simulink model "IMM_UKF"  (R2012b)
settings: Solver=FixedStepDiscrete  StartTime=0.0  StopTime=SimulStop  FixedStep=0.05  RelTol=1e-3
undefined symbols (not defined in the file): mu1_init, mu2_init, PHI, SimulStop, T, T1, xhat_init
libraries: commnoisgen2 x1
settings Model: Creator=DonghanLee  LastModifiedBy=DonghanLee

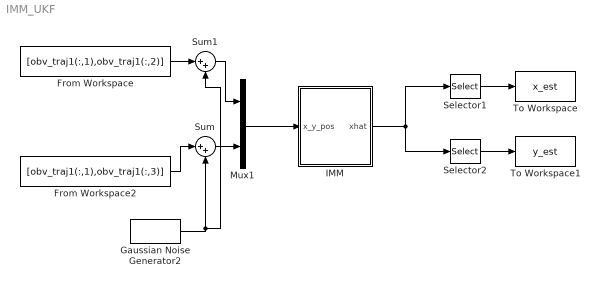
== system IMM_UKF ==
  From Workspace : FromWorkspace  VariableName=[obv_traj1(:,1),obv_traj1(:,2)]  SampleTime=0
  From Workspace2 : FromWorkspace  VariableName=[obv_traj1(:,1),obv_traj1(:,3)]  SampleTime=0
  Gaussian Noise Generator2 : commnoisgen2/Gaussian Noise Generator  m=0  d=noise  s=0  Ts=T  frameBased=off  sampPerFrame=1  orient=off  outDataType=double
  IMM : Subsystem
  Mux1 : Mux  Inputs=2
  Selector1 : Selector  InputPortWidth=5  IndexOptions=Index vector (dialog)  Indices=[1 2]  OutputSizes=1
  Selector2 : Selector  InputPortWidth=5  IndexOptions=Index vector (dialog)  Indices=[3 4]  OutputSizes=1
  Sum : Sum  Inputs=|++
  Sum1 : Sum  Inputs=|++
  To Workspace : ToWorkspace  VariableName=x_est  SampleTime=-1
  To Workspace1 : ToWorkspace  VariableName=y_est  SampleTime=-1
  wires:
  Mux1/1 -> IMM/1(x_y_pos)
  Gaussian Noise Generator2/1 -> Sum1/2, Sum/2
  From Workspace2/1 -> Sum/1
  Sum/1 -> Mux1/2
  From Workspace/1 -> Sum1/1
  Sum1/1 -> Mux1/1
  IMM/1(xhat) -> Selector2/1, Selector1/1
  Selector1/1 -> To Workspace/1
  Selector2/1 -> To Workspace1/1

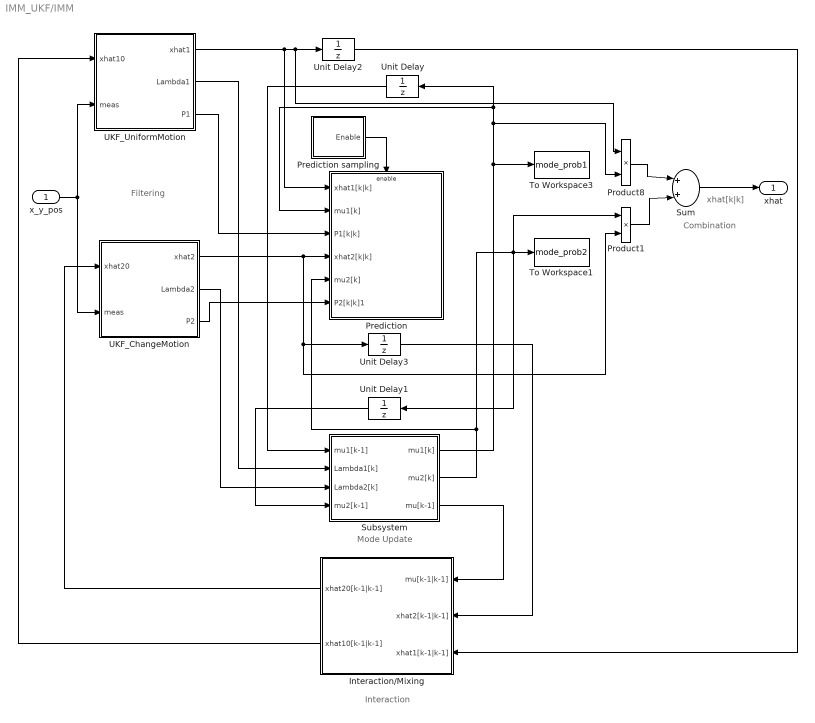
== system IMM_UKF/IMM ==
  note: Mode Update
  note: Interaction
  note: Filtering
  note: xhat[k|k]
  note: Combination
  x_y_pos : Inport
  Interaction/Mixing : Subsystem
  Prediction : Subsystem
  Prediction sampling : Subsystem
  Product1 : Product  SaturateOnIntegerOverflow=on  OutDataTypeStr=Inherit: Same as first input
  Product8 : Product  SaturateOnIntegerOverflow=on  OutDataTypeStr=Inherit: Same as first input
  Subsystem : Subsystem
  Sum : Sum  Inputs=|++|  SaturateOnIntegerOverflow=on
  To Workspace1 : ToWorkspace  VariableName=mode_prob2  SampleTime=-1
  To Workspace3 : ToWorkspace  VariableName=mode_prob1  SampleTime=-1
  UKF_ChangeMotion : Subsystem
  UKF_UniformMotion : Subsystem
  Unit Delay : UnitDelay  InitialCondition=mu1_init  SampleTime=-1
  Unit Delay1 : UnitDelay  InitialCondition=mu2_init  SampleTime=-1
  Unit Delay2 : UnitDelay  InitialCondition=xhat_init  SampleTime=-1
  Unit Delay3 : UnitDelay  InitialCondition=xhat_init  SampleTime=-1
  xhat : Outport
  wires:
  Product8/1 -> Sum/1
  Product1/1 -> Sum/2
  UKF_ChangeMotion/1(xhat2) -> Product1/2, Unit Delay3/1, Prediction/4(xhat2[k|k])
  Subsystem/3(mu[k-1]) -> Interaction/Mixing/1(mu[k-1|k-1])
  Interaction/Mixing/1(xhat20[k-1|k-1]) -> UKF_ChangeMotion/1(xhat20)
  Interaction/Mixing/2(xhat10[k-1|k-1]) -> UKF_UniformMotion/1(xhat10)
  Sum/1 -> xhat/1
  Unit Delay/1 -> Subsystem/1(mu1[k-1])
  Unit Delay1/1 -> Subsystem/4(mu2[k-1])
  Unit Delay3/1 -> Interaction/Mixing/2(xhat2[k-1|k-1])
  Unit Delay2/1 -> Interaction/Mixing/3(xhat1[k-1|k-1])
  x_y_pos/1 -> UKF_UniformMotion/2(meas), UKF_ChangeMotion/2(meas)
  UKF_UniformMotion/1(xhat1) -> Prediction/1(xhat1[k|k]), Product8/1, Unit Delay2/1
  UKF_UniformMotion/2(Lambda1) -> Subsystem/2(Lambda1[k])
  UKF_ChangeMotion/2(Lambda2) -> Subsystem/3(Lambda2[k])
  Subsystem/1(mu1[k]) -> To Workspace3/1, Product8/2, Unit Delay/1, Prediction/2("mu1[k] ")
  Subsystem/2(mu2[k]) -> Product1/1, To Workspace1/1, Unit Delay1/1, Prediction/5(mu2[k])
  Prediction sampling/1(Enable) -> Prediction/Enable
  UKF_UniformMotion/3(P1) -> Prediction/3(P1[k|k])
  UKF_ChangeMotion/3(P2) -> Prediction/6(P2[k|k]1)

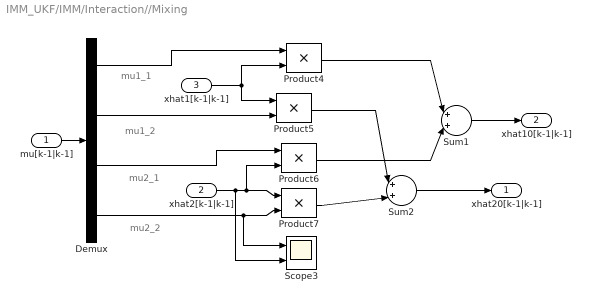
== system IMM_UKF/IMM/Interaction//Mixing ==
  note: mu1_1
  note: mu1_2
  note: mu2_1
  note: mu2_2
  mu[k-1|k-1] : Inport
  xhat2[k-1|k-1] : Inport  Port=2
  xhat1[k-1|k-1] : Inport  Port=3
  Demux : Demux
  Product{4..7} (4 alike) : Product  SaturateOnIntegerOverflow=on  OutDataTypeStr=Inherit: Same as first input
  Scope3 : Scope  NumInputPorts=2
      settings: TimeRange=10  YMin=-5~-5  YMax=5~5  SaveName=ScopeData7
  Sum1 : Sum  Inputs=|++|  SaturateOnIntegerOverflow=on
  Sum2 : Sum  Inputs=|++|  SaturateOnIntegerOverflow=on
  xhat20[k-1|k-1] : Outport
  xhat10[k-1|k-1] : Outport  Port=2
  wires:
  Demux/2 -> Product5/2
  Demux/4 -> Scope3/1, Product7/2
  Product4/1 -> Sum1/1
  Product6/1 -> Sum1/2
  xhat1[k-1|k-1]/1 -> Product4/2, Product5/1
  Demux/1 -> Product4/1
  Demux/3 -> Product6/1
  xhat2[k-1|k-1]/1 -> Scope3/2, Product6/2, Product7/1
  Product5/1 -> Sum2/1
  Product7/1 -> Sum2/2
  Sum2/1 -> xhat20[k-1|k-1]/1
  mu[k-1|k-1]/1 -> Demux/1
  Sum1/1 -> xhat10[k-1|k-1]/1

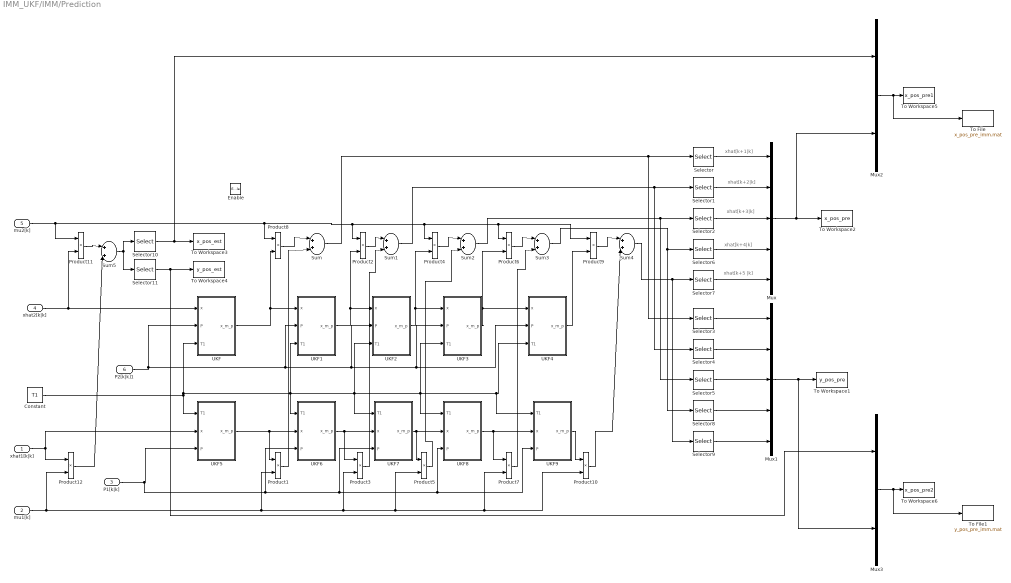
== system IMM_UKF/IMM/Prediction ==
  note: xhat[k+4|k]
  note: xhat[k+3|k]
  note: xhat[k+1|k]
  note: xhat[k+2|k]
  note: xhat[k+5 |k]
  xhat1[k|k] : Inport
  "mu1[k] " : Inport  Port=2
  P1[k|k] : Inport  Port=3
  xhat2[k|k] : Inport  Port=4
  mu2[k] : Inport  Port=5
  P2[k|k]1 : Inport  Port=6
  Enable : EnablePort
  Constant : Constant  Value=T1
  Mux : Mux  Inputs=5
  Mux1 : Mux  Inputs=5
  Mux2 : Mux  Inputs=2
  Mux3 : Mux  Inputs=2
  Product{1..12} (12 alike) : Product  SaturateOnIntegerOverflow=on  OutDataTypeStr=Inherit: Same as first input
  Selector{,1..2,6..7,10} (6 alike) : Selector  InputPortWidth=5  IndexOptions=Index vector (dialog)  Indices=[1]  OutputSizes=1
  Selector{3..5,8..9,11} (6 alike) : Selector  InputPortWidth=5  IndexOptions=Index vector (dialog)  Indices=[3]  OutputSizes=1
  Sum{,1..5} (6 alike) : Sum  Inputs=|++|  SaturateOnIntegerOverflow=on
  To File : ToFile  Filename=x_pos_pre_imm.mat  MatrixName=x_pos_pre_imm
  To File1 : ToFile  Filename=y_pos_pre_imm.mat  MatrixName=y_pos_pre_imm
  To Workspace1 : ToWorkspace  VariableName=y_pos_pre  SampleTime=-1
  To Workspace2 : ToWorkspace  VariableName=x_pos_pre  SampleTime=-1
  To Workspace3 : ToWorkspace  VariableName=x_pos_est  SampleTime=-1
  To Workspace4 : ToWorkspace  VariableName=y_pos_est  SampleTime=-1
  To Workspace5 : ToWorkspace  VariableName=x_pos_pre1  SampleTime=-1
  To Workspace6 : ToWorkspace  VariableName=x_pos_pre2  SampleTime=-1
  UKF : MATLAB Function  TreatAsAtomicUnit=on
  UKF1 : MATLAB Function  TreatAsAtomicUnit=on
  UKF2 : MATLAB Function  TreatAsAtomicUnit=on
  UKF3 : MATLAB Function  TreatAsAtomicUnit=on
  UKF4 : MATLAB Function  TreatAsAtomicUnit=on
  UKF5 : MATLAB Function  TreatAsAtomicUnit=on
  UKF6 : MATLAB Function  TreatAsAtomicUnit=on
  UKF7 : MATLAB Function  TreatAsAtomicUnit=on
  UKF8 : MATLAB Function  TreatAsAtomicUnit=on
  UKF9 : MATLAB Function  TreatAsAtomicUnit=on
  wires:
  xhat1[k|k]/1 -> UKF5/2(x), Product12/1
  UKF/1(x_m_p) -> Product8/2, UKF1/1(x)
  Product8/1 -> Sum/1
  UKF1/1(x_m_p) -> Product2/2, UKF2/1(x)
  Product2/1 -> Sum1/1
  UKF2/1(x_m_p) -> UKF3/1(x), Product4/2
  UKF7/1(x_m_p) -> UKF8/2(x), Product5/1
  Product4/1 -> Sum2/1
  Mux/1 -> Mux2/2, To Workspace2/1
  Mux1/1 -> Mux3/2, To Workspace1/1
  UKF5/1(x_m_p) -> Product1/1, UKF6/2(x)
  UKF6/1(x_m_p) -> Product3/1, UKF7/2(x)
  UKF3/1(x_m_p) -> UKF4/1(x), Product6/2
  UKF8/1(x_m_p) -> Product7/1, UKF9/2(x)
  Product6/1 -> Sum3/1
  mu2[k]/1 -> Product11/1, Product8/1, Product9/1, Product6/1, Product4/1, Product2/1
  "mu1[k] "/1 -> Product12/2, Product1/2, Product10/2, Product7/2, Product5/2, Product3/2
  UKF4/1(x_m_p) -> Product9/2
  UKF9/1(x_m_p) -> Product10/1
  Product9/1 -> Sum4/1
  Product10/1 -> Sum4/2
  Selector6/1 -> Mux/4
  Selector2/1 -> Mux/3
  Selector7/1 -> Mux/5
  Selector/1 -> Mux/1
  Selector1/1 -> Mux/2
  Selector3/1 -> Mux1/1
  Selector4/1 -> Mux1/2
  Selector5/1 -> Mux1/3
  Selector8/1 -> Mux1/4
  Selector9/1 -> Mux1/5
  Sum/1 -> Selector/1, Selector3/1
  Sum1/1 -> Selector4/1, Selector1/1
  Sum2/1 -> Selector5/1, Selector2/1
  Sum3/1 -> Selector8/1, Selector6/1
  Sum4/1 -> Selector9/1, Selector7/1
  xhat2[k|k]/1 -> Product11/2, UKF/1(x)
  Product11/1 -> Sum5/1
  Product12/1 -> Sum5/2
  Sum5/1 -> Selector11/1, Selector10/1
  Selector10/1 -> Mux2/1, To Workspace3/1
  Selector11/1 -> Mux3/1, To Workspace4/1
  Mux2/1 -> To File/1, To Workspace5/1
  Mux3/1 -> To Workspace6/1, To File1/1
  P2[k|k]1/1 -> UKF/2(P), UKF1/2(P), UKF2/2(P), UKF4/2(P), UKF3/2(P)
  Constant/1 -> UKF6/1(T1), UKF7/1(T1), UKF8/1(T1), UKF3/3(T1), UKF9/1(T1), UKF4/3(T1), UKF2/3(T1), UKF1/3(T1), UKF/3(T1), UKF5/1(T1)
  P1[k|k]/1 -> UKF8/3(P), UKF9/3(P), UKF7/3(P), UKF6/3(P), UKF5/3(P)
  Product1/1 -> Sum/2
  Product3/1 -> Sum1/2
  Product5/1 -> Sum2/2
  Product7/1 -> Sum3/2

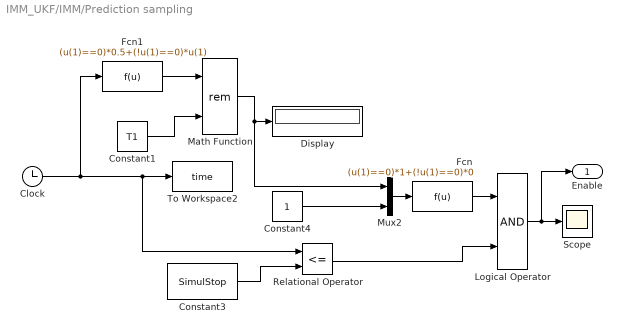
== system IMM_UKF/IMM/Prediction sampling ==
  Clock : Clock
  Constant1 : Constant  Value=T1
  Constant3 : Constant  Value=SimulStop
  Constant4 : Constant
  Display : Display
  Fcn : Fcn  Expr=(u(1)==0)*1+(!u(1)==0)*0
  Fcn1 : Fcn  Expr=(u(1)==0)*0.5+(!u(1)==0)*u(1)
  Logical Operator : Logic  AllPortsSameDT=off  OutDataTypeStr=boolean
  Math Function : Math  Operator=rem  SaturateOnIntegerOverflow=on
  Mux2 : Mux  Inputs=2
  Relational Operator : RelationalOperator  Operator=<=  OutDataTypeStr=boolean
  Scope : Scope
      settings: SaveName=ScopeData2
  To Workspace2 : ToWorkspace  VariableName=time  SampleTime=-1
  Enable : Outport
  wires:
  Clock/1 -> Fcn1/1, Relational Operator/1, To Workspace2/1
  Constant1/1 -> Math Function/2
  Math Function/1 -> Mux2/1, Display/1
  Logical Operator/1 -> Enable/1, Scope/1
  Fcn/1 -> Logical Operator/1
  Relational Operator/1 -> Logical Operator/2
  Constant3/1 -> Relational Operator/2
  Constant4/1 -> Mux2/2
  Mux2/1 -> Fcn/1
  Fcn1/1 -> Math Function/1

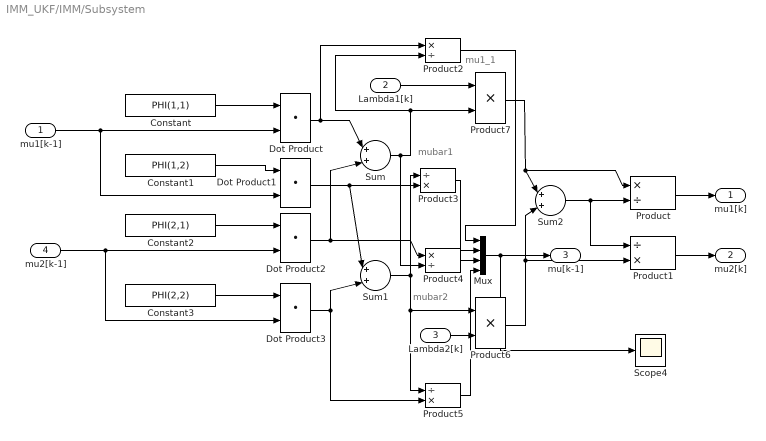
== system IMM_UKF/IMM/Subsystem ==
  note: mubar1
  note: mubar2
  note: mu1_1
  mu1[k-1] : Inport
  Lambda1[k] : Inport  Port=2
  Lambda2[k] : Inport  Port=3
  mu2[k-1] : Inport  Port=4
  Constant : Constant  Value=PHI(1,1)
  Constant1 : Constant  Value=PHI(1,2)
  Constant2 : Constant  Value=PHI(2,1)
  Constant3 : Constant  Value=PHI(2,2)
  Dot Product{,1..3} (4 alike) : DotProduct  InputSameDT=on  OutDataTypeStr=Inherit: Inherit via internal rule
  Mux : Mux
  Product : Product  Inputs=*/  SaturateOnIntegerOverflow=on  OutDataTypeStr=Inherit: Same as first input
  Product1 : Product  Inputs=/*  SaturateOnIntegerOverflow=on  OutDataTypeStr=Inherit: Same as first input
  Product2 : Product  Inputs=*/  SaturateOnIntegerOverflow=on  OutDataTypeStr=Inherit: Same as first input
  Product3 : Product  Inputs=/*  SaturateOnIntegerOverflow=on  OutDataTypeStr=Inherit: Same as first input
  Product4 : Product  Inputs=*/  SaturateOnIntegerOverflow=on  OutDataTypeStr=Inherit: Same as first input
  Product5 : Product  Inputs=/*  SaturateOnIntegerOverflow=on  OutDataTypeStr=Inherit: Same as first input
  Product6 : Product  SaturateOnIntegerOverflow=on  OutDataTypeStr=Inherit: Same as first input
  Product7 : Product  SaturateOnIntegerOverflow=on  OutDataTypeStr=Inherit: Same as first input
  Scope4 : Scope
      settings: YMin=2.77556e-17  YMax=1  SaveName=ScopeData31
  Sum : Sum  Inputs=|++|  SaturateOnIntegerOverflow=on
  Sum1 : Sum  Inputs=|++|  SaturateOnIntegerOverflow=on
  Sum2 : Sum  Inputs=|++|  SaturateOnIntegerOverflow=on
  mu1[k] : Outport
  mu2[k] : Outport  Port=2
  mu[k-1] : Outport  Port=3
  wires:
  Constant/1 -> Dot Product/1
  Constant1/1 -> Dot Product1/1
  Constant2/1 -> Dot Product2/1
  Constant3/1 -> Dot Product3/1
  mu1[k-1]/1 -> Dot Product/2, Dot Product1/2
  mu2[k-1]/1 -> Dot Product2/2, Dot Product3/2
  Dot Product/1 -> Sum/1, Product2/1
  Dot Product2/1 -> Sum/2, Product4/1
  Dot Product1/1 -> Sum1/1, Product3/2
  Dot Product3/1 -> Sum1/2, Product5/2
  Sum1/1 -> Product5/1, Product6/1, Product3/1
  Sum/1 -> Product2/2, Product7/2, Product4/2
  Lambda1[k]/1 -> Product7/1
  Lambda2[k]/1 -> Product6/2
  Product7/1 -> Sum2/1, Product/1
  Product6/1 -> Sum2/2, Product1/2
  Sum2/1 -> Product/2, Product1/1
  Product/1 -> mu1[k]/1
  Product1/1 -> mu2[k]/1
  Product4/1 -> Mux/3
  Product2/1 -> Mux/1
  Product3/1 -> Mux/2
  Product5/1 -> Mux/4
  Mux/1 -> mu[k-1]/1, Scope4/1

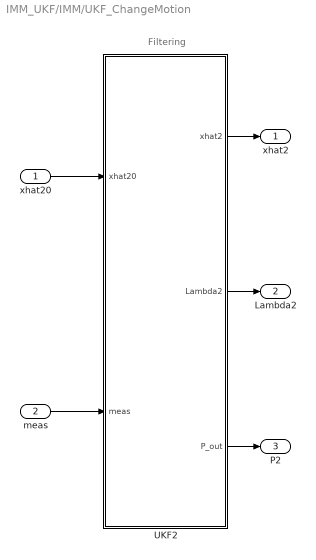
== system IMM_UKF/IMM/UKF_ChangeMotion ==
  note: Filtering
  xhat20 : Inport
  meas : Inport  Port=2
  UKF2 : MATLAB Function  TreatAsAtomicUnit=on
  xhat2 : Outport
  Lambda2 : Outport  Port=2
  P2 : Outport  Port=3
  wires:
  UKF2/2(Lambda2) -> Lambda2/1
  UKF2/1(xhat2) -> xhat2/1
  xhat20/1 -> UKF2/1(xhat20)
  meas/1 -> UKF2/2(meas)
  UKF2/3(P_out) -> P2/1

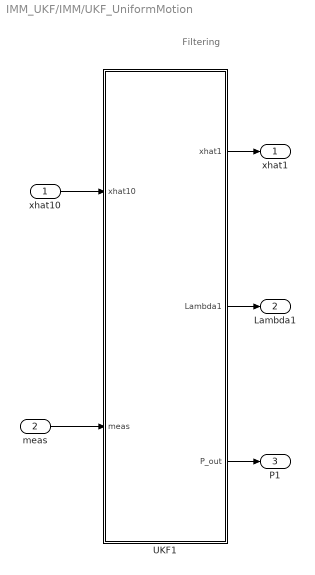
== system IMM_UKF/IMM/UKF_UniformMotion ==
  note: Filtering
  xhat10 : Inport
  meas : Inport  Port=2
  UKF1 : MATLAB Function  TreatAsAtomicUnit=on
  xhat1 : Outport
  Lambda1 : Outport  Port=2
  P1 : Outport  Port=3
  wires:
  meas/1 -> UKF1/2(meas)
  xhat10/1 -> UKF1/1(xhat10)
  UKF1/1(xhat1) -> xhat1/1
  UKF1/2(Lambda1) -> Lambda1/1
  UKF1/3(P_out) -> P1/1

== matlab function IMM_UKF/IMM/UKF_UniformMotion/UKF1 ==
  data: xhat10 input; meas input; xhat1 output; Lambda1 output; P_out output
function [xhat1,Lambda1,P_out] = UKF1(xhat10,meas)
% Define parametersInitialization
T=0.05; % Sampling time [s]
L=5; % Dimension of state vector
% Scaling Factors & Weights
alpha=0.001;                                 %default, tunable
kappa=0;                                       %default, tunable
beta=2;                                     %default, tunable

lambda=alpha^2*(L+kappa)-L;                    %scaling factor
c=L+lambda;                                 %scaling factor
% Wm=[lambda/c 0.5/c*ones(1,2*L)];           %weights for means
% Wc=Wm;
% Wc(1)=Wc(1)+(1-alpha^2+beta);               %weights for covariance

Wm = ones(2*L + 1,1)*1/(2*(L+lambda));
Wc = Wm;
Wm(1) = lambda/(lambda+L);
Wc(1) = lambda/(lambda+L) + 1 - alpha^2 + beta;
c=sqrt(c);

H = [1 0 0 0 0;
     0 0 1 0 0];

% Initialize
persistent P1 W1 V1
if isempty(P1)

% meas_noise1 = 0.5; 
% a_process_noise = 5*10^(-3); 
% w_process_noise = 5*10^(-3);     

% New Feezed value
meas_noise1 = 1.5; 
a_process_noise = 1.5*10^(-2); 
w_process_noise = 1.5*10^(-2);  

Sv1 = meas_noise1^2;
Sw1 = a_process_noise^2;
Sw2 = w_process_noise^2;
Sw = [Sw1 0 0;0 Sw1 0;0 0 Sw2];
%Bw = [0.5*T^2 0 0;T 0 0;0 0.5*T^2 0;0 T 0;0 0 T];

Bw = [T 0 0;1 0 0;0 T 0;0 1 0;0 0 1];

Dw = eye(2);
W1 = Bw*Sw*Bw';
V1 = Dw*Sv1*Dw';

P1 = eye(5,5);
% x = zeros(L, 2*L+1);
% x(:,1) = [meas(1,1);10^(-5);meas(2,1);0;10^(-5)];
%x(:,1) = [meas(1,1);10;meas(2,1);0;10^(-5)];

%y = zeros(L, 2*L+1);
end
% Generate sigma points
x=xhat10;
sP = chol(P1,'lower');
chi_p = [x(:,1) x(:,1)*ones(1,L)+c*sP x(:,1)*ones(1,L)-c*sP];

% Prediction 
    chi_m = zeros(L,2*L+1);
    for i=1:2*L+1        
%         chi_m(1,i) = chi_p(1,i)+ chi_p(2,i)*sin(chi_p(5,i)*T)/chi_p(5,i)-chi_p(4,i)*(1-cos(chi_p(5,i)*T))/chi_p(5,i);
%         chi_m(2,i) = cos(chi_p(5,i)*T)*chi_p(2,i)-sin(chi_p(5,i)*T)*chi_p(4,i);
%         chi_m(3,i) = chi_p(2,i)*(1-cos(chi_p(5,i)*T))/chi_p(5,i)+chi_p(3,i)+chi_p(4,i)*sin(chi_p(5,i)*T)/chi_p(5,i);
%         chi_m(4,i) = chi_p(2,i)*sin(chi_p(5,i)*T)+chi_p(4,i)*cos(chi_p(5,i)*T);
%         chi_m(5,i) = chi_p(5,i);
        
        chi_m(1,i) = chi_p(1,i)+ chi_p(2,i)*T;
        chi_m(2,i) = chi_p(2,i);
        chi_m(3,i) = chi_p(3,i)+ chi_p(4,i)*T;
        chi_m(4,i) = chi_p(4,i);
        chi_m(5,i) = 0;
    end        
    x_m = chi_m*Wm;    
    P_m = W1;
    for i=1:2*L+1
        P_m = P_m+Wc(i)*(chi_m(:,i)-x_m)*(chi_m(:,i)-x_m)';
    end
    psi_m = H*chi_m;
    y_m = psi_m*Wm;
    
% Update
    Pyy = V1;
    Pxy = zeros(L,2);
    for i=1:2*L+1
        Pyy = Pyy+Wc(i)*(psi_m(:,i)-y_m)*(psi_m(:,i)-y_m)';
        Pxy = Pxy+Wc(i)*(chi_m(:,i)-x_m)*(psi_m(:,i)-y_m)';
    end
    
    K = Pxy*inv(Pyy);
    xhat1 = x_m + K*(meas - y_m);
    P1 = P_m-K*Pyy*K';
    
    innov = meas - y_m;  % Innovation
    Lambda1 = 1/sqrt((2*pi)^2*Pyy(1,1)*Pyy(2,2))*expm(-1/2*(innov'*inv(Pyy)*innov)); % Likelihood function
% Post the results
% x_pos = x(1,1);
% x_vel = x(2,1);
% y_pos = x(3,1);
% y_vel = x(4,1);
% turn_rate = x(5,1);
P_out=P1;   
c_out = c;
Wm_out = Wm;

== matlab function IMM_UKF/IMM/Prediction/UKF ==
  data: x input; P input; T1 input; x_m_p output
function x_m_p  = UKF_pred2(x,P,T1)
L=5; % Dimension of state vector
% Scaling Factors & Weights
alpha=0.001;                                 %default, tunable
kappa=0;                                       %default, tunable
beta=2;                                     %default, tunable

lambda=alpha^2*(L+kappa)-L;                    %scaling factor
c=L+lambda;                                 %scaling factor
% Wm=[lambda/c 0.5/c*ones(1,2*L)];           %weights for means
% Wc=Wm;
% Wc(1)=Wc(1)+(1-alpha^2+beta);               %weights for covariance

Wm = ones(2*L + 1,1)*1/(2*(L+lambda));
Wc = Wm;
Wm(1) = lambda/(lambda+L);
Wc(1) = lambda/(lambda+L) + 1 - alpha^2 + beta;
c=sqrt(c);

sP = chol(P,'lower');
chi_p = [x(:,1) x(:,1)*ones(1,L)+c*sP x(:,1)*ones(1,L)-c*sP];

% Prediction 
    chi_m_p = zeros(L,2*L+1);
    for i=1:2*L+1        
        chi_m_p(1,i) = chi_p(1,i)+ chi_p(2,i)*sin(chi_p(5,i)*T1)/chi_p(5,i)-chi_p(4,i)*(1-cos(chi_p(5,i)*T1))/chi_p(5,i);
        chi_m_p(2,i) = cos(chi_p(5,i)*T1)*chi_p(2,i)-sin(chi_p(5,i)*T1)*chi_p(4,i);
        chi_m_p(3,i) = chi_p(2,i)*(1-cos(chi_p(5,i)*T1))/chi_p(5,i)+chi_p(3,i)+chi_p(4,i)*sin(chi_p(5,i)*T1)/chi_p(5,i);
        chi_m_p(4,i) = chi_p(2,i)*sin(chi_p(5,i)*T1)+chi_p(4,i)*cos(chi_p(5,i)*T1);
        chi_m_p(5,i) = chi_p(5,i);
    end        
    x_m_p = chi_m_p*Wm;

== matlab function IMM_UKF/IMM/Prediction/UKF1 ==
  data: x input; P input; T1 input; x_m_p output
function x_m_p  = UKF_pred2(x,P,T1)
L=5; % Dimension of state vector
% Scaling Factors & Weights
alpha=0.001;                                 %default, tunable
kappa=0;                                       %default, tunable
beta=2;                                     %default, tunable

lambda=alpha^2*(L+kappa)-L;                    %scaling factor
c=L+lambda;                                 %scaling factor
% Wm=[lambda/c 0.5/c*ones(1,2*L)];           %weights for means
% Wc=Wm;
% Wc(1)=Wc(1)+(1-alpha^2+beta);               %weights for covariance

Wm = ones(2*L + 1,1)*1/(2*(L+lambda));
Wc = Wm;
Wm(1) = lambda/(lambda+L);
Wc(1) = lambda/(lambda+L) + 1 - alpha^2 + beta;
c=sqrt(c);

sP = chol(P,'lower');
chi_p = [x(:,1) x(:,1)*ones(1,L)+c*sP x(:,1)*ones(1,L)-c*sP];

% Prediction 
    chi_m_p = zeros(L,2*L+1);
    for i=1:2*L+1        
        chi_m_p(1,i) = chi_p(1,i)+ chi_p(2,i)*sin(chi_p(5,i)*T1)/chi_p(5,i)-chi_p(4,i)*(1-cos(chi_p(5,i)*T1))/chi_p(5,i);
        chi_m_p(2,i) = cos(chi_p(5,i)*T1)*chi_p(2,i)-sin(chi_p(5,i)*T1)*chi_p(4,i);
        chi_m_p(3,i) = chi_p(2,i)*(1-cos(chi_p(5,i)*T1))/chi_p(5,i)+chi_p(3,i)+chi_p(4,i)*sin(chi_p(5,i)*T1)/chi_p(5,i);
        chi_m_p(4,i) = chi_p(2,i)*sin(chi_p(5,i)*T1)+chi_p(4,i)*cos(chi_p(5,i)*T1);
        chi_m_p(5,i) = chi_p(5,i);
    end        
    x_m_p = chi_m_p*Wm;

== matlab function IMM_UKF/IMM/Prediction/UKF2 ==
  data: x input; P input; T1 input; x_m_p output
function x_m_p  = UKF_pred2(x,P,T1)
L=5; % Dimension of state vector
% Scaling Factors & Weights
alpha=0.001;                                 %default, tunable
kappa=0;                                       %default, tunable
beta=2;                                     %default, tunable

lambda=alpha^2*(L+kappa)-L;                    %scaling factor
c=L+lambda;                                 %scaling factor
% Wm=[lambda/c 0.5/c*ones(1,2*L)];           %weights for means
% Wc=Wm;
% Wc(1)=Wc(1)+(1-alpha^2+beta);               %weights for covariance

Wm = ones(2*L + 1,1)*1/(2*(L+lambda));
Wc = Wm;
Wm(1) = lambda/(lambda+L);
Wc(1) = lambda/(lambda+L) + 1 - alpha^2 + beta;
c=sqrt(c);

sP = chol(P,'lower');
chi_p = [x(:,1) x(:,1)*ones(1,L)+c*sP x(:,1)*ones(1,L)-c*sP];

% Prediction 
    chi_m_p = zeros(L,2*L+1);
    for i=1:2*L+1        
        chi_m_p(1,i) = chi_p(1,i)+ chi_p(2,i)*sin(chi_p(5,i)*T1)/chi_p(5,i)-chi_p(4,i)*(1-cos(chi_p(5,i)*T1))/chi_p(5,i);
        chi_m_p(2,i) = cos(chi_p(5,i)*T1)*chi_p(2,i)-sin(chi_p(5,i)*T1)*chi_p(4,i);
        chi_m_p(3,i) = chi_p(2,i)*(1-cos(chi_p(5,i)*T1))/chi_p(5,i)+chi_p(3,i)+chi_p(4,i)*sin(chi_p(5,i)*T1)/chi_p(5,i);
        chi_m_p(4,i) = chi_p(2,i)*sin(chi_p(5,i)*T1)+chi_p(4,i)*cos(chi_p(5,i)*T1);
        chi_m_p(5,i) = chi_p(5,i);
    end        
    x_m_p = chi_m_p*Wm;

== matlab function IMM_UKF/IMM/Prediction/UKF3 ==
  data: x input; P input; T1 input; x_m_p output
function x_m_p  = UKF_pred2(x,P,T1)
L=5; % Dimension of state vector
% Scaling Factors & Weights
alpha=0.001;                                 %default, tunable
kappa=0;                                       %default, tunable
beta=2;                                     %default, tunable

lambda=alpha^2*(L+kappa)-L;                    %scaling factor
c=L+lambda;                                 %scaling factor
% Wm=[lambda/c 0.5/c*ones(1,2*L)];           %weights for means
% Wc=Wm;
% Wc(1)=Wc(1)+(1-alpha^2+beta);               %weights for covariance

Wm = ones(2*L + 1,1)*1/(2*(L+lambda));
Wc = Wm;
Wm(1) = lambda/(lambda+L);
Wc(1) = lambda/(lambda+L) + 1 - alpha^2 + beta;
c=sqrt(c);

sP = chol(P,'lower');
chi_p = [x(:,1) x(:,1)*ones(1,L)+c*sP x(:,1)*ones(1,L)-c*sP];

% Prediction 
    chi_m_p = zeros(L,2*L+1);
    for i=1:2*L+1        
        chi_m_p(1,i) = chi_p(1,i)+ chi_p(2,i)*sin(chi_p(5,i)*T1)/chi_p(5,i)-chi_p(4,i)*(1-cos(chi_p(5,i)*T1))/chi_p(5,i);
        chi_m_p(2,i) = cos(chi_p(5,i)*T1)*chi_p(2,i)-sin(chi_p(5,i)*T1)*chi_p(4,i);
        chi_m_p(3,i) = chi_p(2,i)*(1-cos(chi_p(5,i)*T1))/chi_p(5,i)+chi_p(3,i)+chi_p(4,i)*sin(chi_p(5,i)*T1)/chi_p(5,i);
        chi_m_p(4,i) = chi_p(2,i)*sin(chi_p(5,i)*T1)+chi_p(4,i)*cos(chi_p(5,i)*T1);
        chi_m_p(5,i) = chi_p(5,i);
    end        
    x_m_p = chi_m_p*Wm;

== matlab function IMM_UKF/IMM/Prediction/UKF4 ==
  data: x input; P input; T1 input; x_m_p output
function x_m_p  = UKF_pred2(x,P,T1)
L=5; % Dimension of state vector
% Scaling Factors & Weights
alpha=0.001;                                 %default, tunable
kappa=0;                                       %default, tunable
beta=2;                                     %default, tunable

lambda=alpha^2*(L+kappa)-L;                    %scaling factor
c=L+lambda;                                 %scaling factor
% Wm=[lambda/c 0.5/c*ones(1,2*L)];           %weights for means
% Wc=Wm;
% Wc(1)=Wc(1)+(1-alpha^2+beta);               %weights for covariance

Wm = ones(2*L + 1,1)*1/(2*(L+lambda));
Wc = Wm;
Wm(1) = lambda/(lambda+L);
Wc(1) = lambda/(lambda+L) + 1 - alpha^2 + beta;
c=sqrt(c);

sP = chol(P,'lower');
chi_p = [x(:,1) x(:,1)*ones(1,L)+c*sP x(:,1)*ones(1,L)-c*sP];

% Prediction 
    chi_m_p = zeros(L,2*L+1);
    for i=1:2*L+1        
        chi_m_p(1,i) = chi_p(1,i)+ chi_p(2,i)*sin(chi_p(5,i)*T1)/chi_p(5,i)-chi_p(4,i)*(1-cos(chi_p(5,i)*T1))/chi_p(5,i);
        chi_m_p(2,i) = cos(chi_p(5,i)*T1)*chi_p(2,i)-sin(chi_p(5,i)*T1)*chi_p(4,i);
        chi_m_p(3,i) = chi_p(2,i)*(1-cos(chi_p(5,i)*T1))/chi_p(5,i)+chi_p(3,i)+chi_p(4,i)*sin(chi_p(5,i)*T1)/chi_p(5,i);
        chi_m_p(4,i) = chi_p(2,i)*sin(chi_p(5,i)*T1)+chi_p(4,i)*cos(chi_p(5,i)*T1);
        chi_m_p(5,i) = chi_p(5,i);
    end        
    x_m_p = chi_m_p*Wm;

== matlab function IMM_UKF/IMM/UKF_ChangeMotion/UKF2 ==
  data: xhat20 input; meas input; xhat2 output; Lambda2 output; P_out output
function [xhat2,Lambda2,P_out] = UKF2(xhat20,meas)
% Define parametersInitialization
T=0.05; % Sampling time [s]
L=5; % Dimension of state vector
% Scaling Factors & Weights
alpha=0.001;                                 %default, tunable
kappa=0;                                       %default, tunable
beta=2;                                     %default, tunable

lambda=alpha^2*(L+kappa)-L;                    %scaling factor
c=L+lambda;                                 %scaling factor
% Wm=[lambda/c 0.5/c*ones(1,2*L)];           %weights for means
% Wc=Wm;
% Wc(1)=Wc(1)+(1-alpha^2+beta);               %weights for covariance

Wm = ones(2*L + 1,1)*1/(2*(L+lambda));
Wc = Wm;
Wm(1) = lambda/(lambda+L);
Wc(1) = lambda/(lambda+L) + 1 - alpha^2 + beta;
c=sqrt(c);

H = [1 0 0 0 0;
     0 0 1 0 0];

% Initialize
persistent P2 W2 V2
if isempty(P2)
% meas_noise1 = 0.5; 
% a_process_noise = 5*10^(-3); 
% w_process_noise = 5*10^(-4);  

meas_noise1 = 1.5;     % New freezed value
a_process_noise = 1.5*10^(-2); 
w_process_noise = 1.5*10^(-3); 

Sv1 = meas_noise1^2;
Sw1 = a_process_noise^2;
Sw2 = w_process_noise^2;
Sw = [Sw1 0 0;0 Sw1 0;0 0 Sw2];
%Bw = [0.5*T^2 0 0;T 0 0;0 0.5*T^2 0;0 T 0;0 0 T];

Bw = [T 0 0;1 0 0;0 T 0;0 1 0;0 0 1];

Dw = eye(2);
W2 = Bw*Sw*Bw';
V2 = Dw*Sv1*Dw';

P2 = eye(5,5);
% x = zeros(L, 2*L+1);
% x(:,1) = [meas(1,1);10^(-5);meas(2,1);0;10^(-5)];
%x(:,1) = [meas(1,1);10;meas(2,1);0;10^(-5)];

%y = zeros(L, 2*L+1);
end
% Generate sigma points
x=xhat20;
sP = chol(P2,'lower');
chi_p = [x(:,1) x(:,1)*ones(1,L)+c*sP x(:,1)*ones(1,L)-c*sP];

% Prediction 
    chi_m = zeros(L,2*L+1);
    for i=1:2*L+1        
        chi_m(1,i) = chi_p(1,i)+ chi_p(2,i)*sin(chi_p(5,i)*T)/chi_p(5,i)-chi_p(4,i)*(1-cos(chi_p(5,i)*T))/chi_p(5,i);
        chi_m(2,i) = cos(chi_p(5,i)*T)*chi_p(2,i)-sin(chi_p(5,i)*T)*chi_p(4,i);
        chi_m(3,i) = chi_p(2,i)*(1-cos(chi_p(5,i)*T))/chi_p(5,i)+chi_p(3,i)+chi_p(4,i)*sin(chi_p(5,i)*T)/chi_p(5,i);
        chi_m(4,i) = chi_p(2,i)*sin(chi_p(5,i)*T)+chi_p(4,i)*cos(chi_p(5,i)*T);
        chi_m(5,i) = chi_p(5,i);
    end        
    x_m = chi_m*Wm;    
    P_m = W2;
    for i=1:2*L+1
        P_m = P_m+Wc(i)*(chi_m(:,i)-x_m)*(chi_m(:,i)-x_m)';
    end
    psi_m = H*chi_m;
    y_m = psi_m*Wm;
    
% Update
    Pyy = V2;
    Pxy = zeros(L,2);
    for i=1:2*L+1
        Pyy = Pyy+Wc(i)*(psi_m(:,i)-y_m)*(psi_m(:,i)-y_m)';
        Pxy = Pxy+Wc(i)*(chi_m(:,i)-x_m)*(psi_m(:,i)-y_m)';
    end
    
    K = Pxy*inv(Pyy);
    xhat2 = x_m + K*(meas - y_m);
    P2 = P_m-K*Pyy*K';
    
    innov = meas - y_m;  % Innovation
    Lambda2 = 1/sqrt((2*pi)^2*Pyy(1,1)*Pyy(2,2))*expm(-1/2*(innov'*inv(Pyy)*innov)); % Likelihood function
% Post the results
% x_pos = x(1,1);
% x_vel = x(2,1);
% y_pos = x(3,1);
% y_vel = x(4,1);
% turn_rate = x(5,1);
P_out=P2;   
c_out = c;
Wm_out = Wm;

== matlab function IMM_UKF/IMM/Prediction/UKF5 ==
  data: T1 input; x input; P input; x_m_p output
function x_m_p  = UKF_pred1(T1,x,P)
L=5; % Dimension of state vector
% Scaling Factors & Weights
alpha=0.001;                                 %default, tunable
kappa=0;                                       %default, tunable
beta=2;                                     %default, tunable

lambda=alpha^2*(L+kappa)-L;                    %scaling factor
c=L+lambda;                                 %scaling factor
% Wm=[lambda/c 0.5/c*ones(1,2*L)];           %weights for means
% Wc=Wm;
% Wc(1)=Wc(1)+(1-alpha^2+beta);               %weights for covariance

Wm = ones(2*L + 1,1)*1/(2*(L+lambda));
Wc = Wm;
Wm(1) = lambda/(lambda+L);
Wc(1) = lambda/(lambda+L) + 1 - alpha^2 + beta;
c=sqrt(c);

sP = chol(P,'lower');
chi_p = [x(:,1) x(:,1)*ones(1,L)+c*sP x(:,1)*ones(1,L)-c*sP];

% Prediction 
    chi_m_p = zeros(L,2*L+1);
    for i=1:2*L+1        
        chi_m_p(1,i) = chi_p(1,i)+ chi_p(2,i)*T1;
        chi_m_p(2,i) = chi_p(2,i);
        chi_m_p(3,i) = chi_p(3,i)+ chi_p(4,i)*T1;
        chi_m_p(4,i) = chi_p(4,i);
        chi_m_p(5,i) = 0;
    end        
    x_m_p = chi_m_p*Wm;

== matlab function IMM_UKF/IMM/Prediction/UKF6 ==
  data: T1 input; x input; P input; x_m_p output
function x_m_p  = UKF_pred1(T1,x,P)
L=5; % Dimension of state vector
% Scaling Factors & Weights
alpha=0.001;                                 %default, tunable
kappa=0;                                       %default, tunable
beta=2;                                     %default, tunable

lambda=alpha^2*(L+kappa)-L;                    %scaling factor
c=L+lambda;                                 %scaling factor
% Wm=[lambda/c 0.5/c*ones(1,2*L)];           %weights for means
% Wc=Wm;
% Wc(1)=Wc(1)+(1-alpha^2+beta);               %weights for covariance

Wm = ones(2*L + 1,1)*1/(2*(L+lambda));
Wc = Wm;
Wm(1) = lambda/(lambda+L);
Wc(1) = lambda/(lambda+L) + 1 - alpha^2 + beta;
c=sqrt(c);

sP = chol(P,'lower');
chi_p = [x(:,1) x(:,1)*ones(1,L)+c*sP x(:,1)*ones(1,L)-c*sP];

% Prediction 
    chi_m_p = zeros(L,2*L+1);
    for i=1:2*L+1        
        chi_m_p(1,i) = chi_p(1,i)+ chi_p(2,i)*T1;
        chi_m_p(2,i) = chi_p(2,i);
        chi_m_p(3,i) = chi_p(3,i)+ chi_p(4,i)*T1;
        chi_m_p(4,i) = chi_p(4,i);
        chi_m_p(5,i) = 0;
    end        
    x_m_p = chi_m_p*Wm;

== matlab function IMM_UKF/IMM/Prediction/UKF7 ==
  data: T1 input; x input; P input; x_m_p output
function x_m_p  = UKF_pred1(T1,x,P)
L=5; % Dimension of state vector
% Scaling Factors & Weights
alpha=0.001;                                 %default, tunable
kappa=0;                                       %default, tunable
beta=2;                                     %default, tunable

lambda=alpha^2*(L+kappa)-L;                    %scaling factor
c=L+lambda;                                 %scaling factor
% Wm=[lambda/c 0.5/c*ones(1,2*L)];           %weights for means
% Wc=Wm;
% Wc(1)=Wc(1)+(1-alpha^2+beta);               %weights for covariance

Wm = ones(2*L + 1,1)*1/(2*(L+lambda));
Wc = Wm;
Wm(1) = lambda/(lambda+L);
Wc(1) = lambda/(lambda+L) + 1 - alpha^2 + beta;
c=sqrt(c);

sP = chol(P,'lower');
chi_p = [x(:,1) x(:,1)*ones(1,L)+c*sP x(:,1)*ones(1,L)-c*sP];

% Prediction 
    chi_m_p = zeros(L,2*L+1);
    for i=1:2*L+1        
        chi_m_p(1,i) = chi_p(1,i)+ chi_p(2,i)*T1;
        chi_m_p(2,i) = chi_p(2,i);
        chi_m_p(3,i) = chi_p(3,i)+ chi_p(4,i)*T1;
        chi_m_p(4,i) = chi_p(4,i);
        chi_m_p(5,i) = 0;
    end        
    x_m_p = chi_m_p*Wm;

== matlab function IMM_UKF/IMM/Prediction/UKF8 ==
  data: T1 input; x input; P input; x_m_p output
function x_m_p  = UKF_pred1(T1,x,P)
L=5; % Dimension of state vector
% Scaling Factors & Weights
alpha=0.001;                                 %default, tunable
kappa=0;                                       %default, tunable
beta=2;                                     %default, tunable

lambda=alpha^2*(L+kappa)-L;                    %scaling factor
c=L+lambda;                                 %scaling factor
% Wm=[lambda/c 0.5/c*ones(1,2*L)];           %weights for means
% Wc=Wm;
% Wc(1)=Wc(1)+(1-alpha^2+beta);               %weights for covariance

Wm = ones(2*L + 1,1)*1/(2*(L+lambda));
Wc = Wm;
Wm(1) = lambda/(lambda+L);
Wc(1) = lambda/(lambda+L) + 1 - alpha^2 + beta;
c=sqrt(c);

sP = chol(P,'lower');
chi_p = [x(:,1) x(:,1)*ones(1,L)+c*sP x(:,1)*ones(1,L)-c*sP];

% Prediction 
    chi_m_p = zeros(L,2*L+1);
    for i=1:2*L+1        
        chi_m_p(1,i) = chi_p(1,i)+ chi_p(2,i)*T1;
        chi_m_p(2,i) = chi_p(2,i);
        chi_m_p(3,i) = chi_p(3,i)+ chi_p(4,i)*T1;
        chi_m_p(4,i) = chi_p(4,i);
        chi_m_p(5,i) = 0;
    end        
    x_m_p = chi_m_p*Wm;

== matlab function IMM_UKF/IMM/Prediction/UKF9 ==
  data: T1 input; x input; P input; x_m_p output
function x_m_p  = UKF_pred1(T1,x,P)
L=5; % Dimension of state vector
% Scaling Factors & Weights
alpha=0.001;                                 %default, tunable
kappa=0;                                       %default, tunable
beta=2;                                     %default, tunable

lambda=alpha^2*(L+kappa)-L;                    %scaling factor
c=L+lambda;                                 %scaling factor
% Wm=[lambda/c 0.5/c*ones(1,2*L)];           %weights for means
% Wc=Wm;
% Wc(1)=Wc(1)+(1-alpha^2+beta);               %weights for covariance

Wm = ones(2*L + 1,1)*1/(2*(L+lambda));
Wc = Wm;
Wm(1) = lambda/(lambda+L);
Wc(1) = lambda/(lambda+L) + 1 - alpha^2 + beta;
c=sqrt(c);

sP = chol(P,'lower');
chi_p = [x(:,1) x(:,1)*ones(1,L)+c*sP x(:,1)*ones(1,L)-c*sP];

% Prediction 
    chi_m_p = zeros(L,2*L+1);
    for i=1:2*L+1        
        chi_m_p(1,i) = chi_p(1,i)+ chi_p(2,i)*T1;
        chi_m_p(2,i) = chi_p(2,i);
        chi_m_p(3,i) = chi_p(3,i)+ chi_p(4,i)*T1;
        chi_m_p(4,i) = chi_p(4,i);
        chi_m_p(5,i) = 0;
    end        
    x_m_p = chi_m_p*Wm;
